simulink model "position_lqi_controller_v1_sim"  (R2023b)
settings: Solver=ode4  StartTime=0.0  StopTime=2.5  FixedStep=0.001  RelTol=1e-3  EnableMultiTasking=on
undefined symbols (not defined in the file or in its folder): K
libraries: simulink_extras x2
settings Model: ExtModeTrigDuration=10  Creator=paoli  LastModifiedBy=kiraa
settings OptimizationCC: DefaultParameterBehavior=Inlined  EnhancedBackFolding=on  PassReuseOutputArgsAs=Individual arguments  ZeroExternalMemoryAtStartup=off  ZeroInternalMemoryAtStartup=off  MaxStackSize=64  OptimizeBlockOrder=speed  DifferentSizesBufferReuse=on  OptimizationCustomize=off  EfficientTunableParamExpr=on
settings DebuggingCC: ParameterTunabilityLossMsg=error
settings HardwareCC: ProdBitPerPointer=32  ProdBitPerSizeT=32  ProdBitPerPtrDiffT=32  ProdLargestAtomicInteger=Long  ProdLargestAtomicFloat=Double  ProdWordSize=32  ProdLongLongMode=on  ProdHWDeviceType=ARM Compatible->ARM Cortex
settings SFSimCC: MATLABDynamicMemAlloc=off
settings RTWCC: Description=Embedded Coder  SystemTargetFile=ert.tlc  TemplateMakefile=ert_default_tmf  Toolchain=GNU Tools for ARM Embedded Processors
settings CodeAppCC: ForceParamTrailComments=on  IgnoreCustomStorageClasses=off  OperatorAnnotations=on  SimulinkDataObjDesc=on  SFDataObjDesc=on  InsertBlockDesc=on
settings ERTTargetCC: SupportContinuousTime=on  ExtModeTransport=3  ExtModeStaticAlloc=on  ExtModeStaticAllocSize=2000  ExtModeMexFile=ext_xcp  ExtModeIntrfLevel=Level2 - Open  InlinedParameterPlacement=NonHierarchical  ERTCustomFileTemplate=example_file_process.tlc

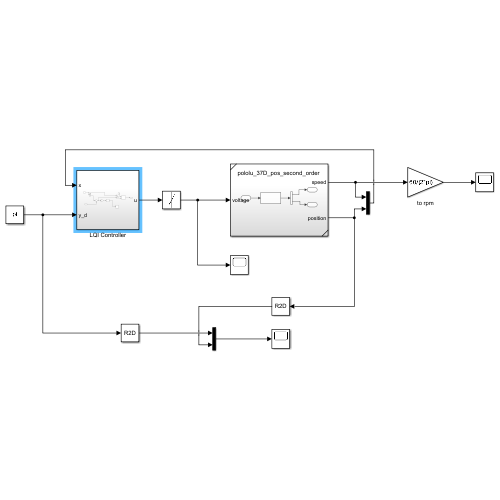
[thumbnail: Simulink's stored preview of the top-level diagram]
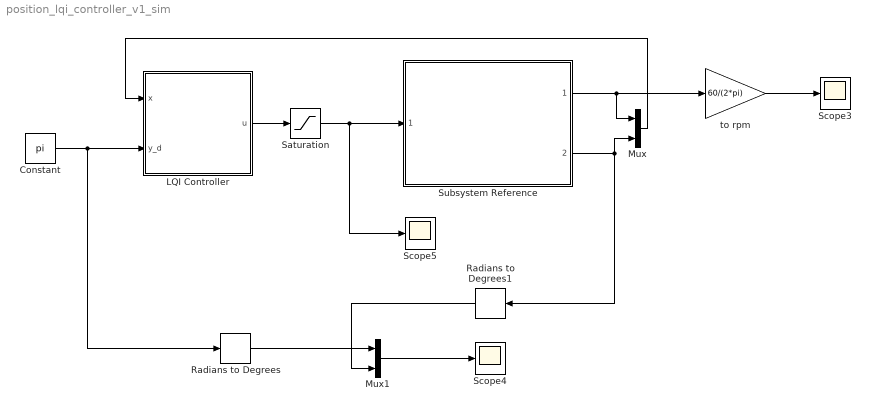
== system position_lqi_controller_v1_sim ==
  Constant : Constant  Value=pi
  LQI Controller : Subsystem
  Mux : Mux  Inputs=2
  Mux1 : Mux  Inputs=2
  Radians to Degrees : simulink_extras/Transformations/Radians to Degrees
  Radians to Degrees1 : simulink_extras/Transformations/Radians to Degrees
  Saturation : Saturate  UpperLimit=12  LowerLimit=-12
  Scope3 : Scope
  Scope4 : Scope
  Scope5 : Scope
  Subsystem Reference : Subsystem  ReferencedSubsystem=pololu_37D_pos_second_order
  to rpm : Gain  Gain=60/(2*pi)
  wires:
  Mux/1 -> LQI Controller/1(x)
  Subsystem Reference/1 -> Mux/1, to rpm/1
  Subsystem Reference/2 -> Radians to Degrees1/1, Mux/2
  to rpm/1 -> Scope3/1
  Constant/1 -> Radians to Degrees/1, LQI Controller/2(y_d)
  Mux1/1 -> Scope4/1
  LQI Controller/1(u) -> Saturation/1
  Saturation/1 -> Scope5/1, Subsystem Reference/1
  Radians to Degrees/1 -> Mux1/1
  Radians to Degrees1/1 -> Mux1/2

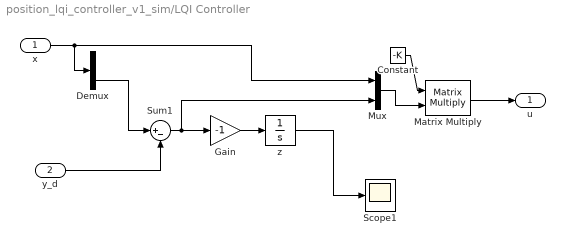
== system position_lqi_controller_v1_sim/LQI Controller ==
  x : Inport
  y_d : Inport  Port=2
  Constant : Constant  Value=-K  VectorParams1D=off
  Demux : Demux  Outputs=2
  Gain : Gain  Gain=-1
  Matrix Multiply : Product  Multiplication=Matrix(*)
  Mux : Mux  Inputs=2
  Scope1 : Scope
  Sum1 : Sum  Inputs=|+-
  z : Integrator
  u : Outport
  wires:
  Constant/1 -> Matrix Multiply/1
  x/1 -> Demux/1, Mux/1
  Mux/1 -> Matrix Multiply/2
  Sum1/1 -> Mux/2, Gain/1
  y_d/1 -> Sum1/2
  z/1 -> Scope1/1
  Demux/2 -> Sum1/1
  Gain/1 -> z/1
  Matrix Multiply/1 -> u/1
